simulink model "Unigo_Simulink1"  (R2023b)
settings: Solver=VariableStepAuto  StartTime=0.0  StopTime=20  RelTol=1e-3
values from neighbouring files (symbols this model uses):
  G_den1 = [1 2 1]    [Unigo_Number12.m]
  G_num1 = [1]    [Unigo_Number12.m]
settings Model: Creator=user  LastModifiedBy=user

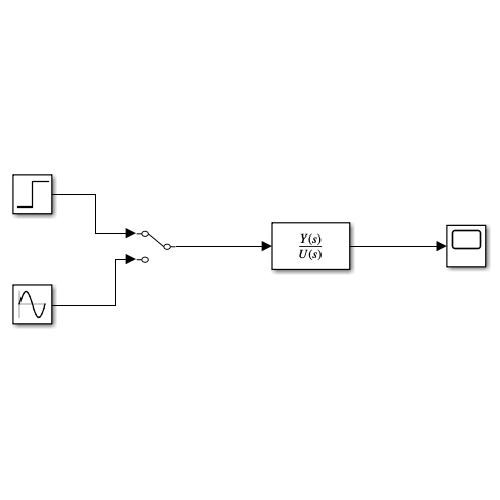
[thumbnail: Simulink's stored preview of the top-level diagram]
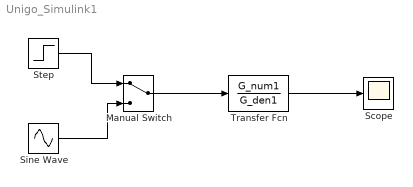
== system Unigo_Simulink1 ==
  Manual Switch : ManualSwitch
  Scope : Scope
  Sine Wave : Sin  SampleTime=0
  Step : Step  Time=0  SampleTime=0
  Transfer Fcn : TransferFcn  Numerator=G_num1  Denominator=G_den1
  wires:
  Step/1 -> Manual Switch/1
  Sine Wave/1 -> Manual Switch/2
  Manual Switch/1 -> Transfer Fcn/1
  Transfer Fcn/1 -> Scope/1
